simulink model "Bike2DOF"  (R2023a)
settings: Solver=VariableStepAuto  StartTime=0.0  StopTime=10.0  RelTol=1e-3
undefined symbols (not defined in the file): Iz, l_f, l_r, m
settings Model: Creator=Tan_Tram  LastModifiedBy=Tan_Tram

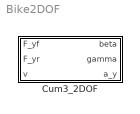
== system Bike2DOF ==
  Cum3_2DOF : Subsystem

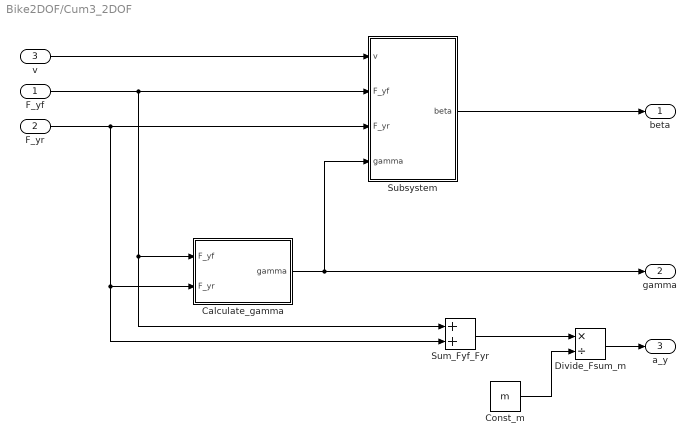
== system Bike2DOF/Cum3_2DOF ==
  F_yf : Inport
  F_yr : Inport  Port=2
  v : Inport  Port=3
  Calculate_gamma : Subsystem
  Const_m : Constant  Value=m
  Divide_Fsum_m : Product  Inputs=*/
  Subsystem : Subsystem
  Sum_Fyf_Fyr : Sum
  beta : Outport
  gamma : Outport  Port=2
  a_y : Outport  Port=3
  wires:
  F_yf/1 -> Subsystem/2(F_yf), Calculate_gamma/1(F_yf), Sum_Fyf_Fyr/1
  F_yr/1 -> Calculate_gamma/2(F_yr), Sum_Fyf_Fyr/2, Subsystem/3(F_yr)
  Const_m/1 -> Divide_Fsum_m/2
  Sum_Fyf_Fyr/1 -> Divide_Fsum_m/1
  Divide_Fsum_m/1 -> a_y/1
  Calculate_gamma/1(gamma) -> Subsystem/4(gamma), gamma/1
  v/1 -> Subsystem/1(v)
  Subsystem/1(beta) -> beta/1

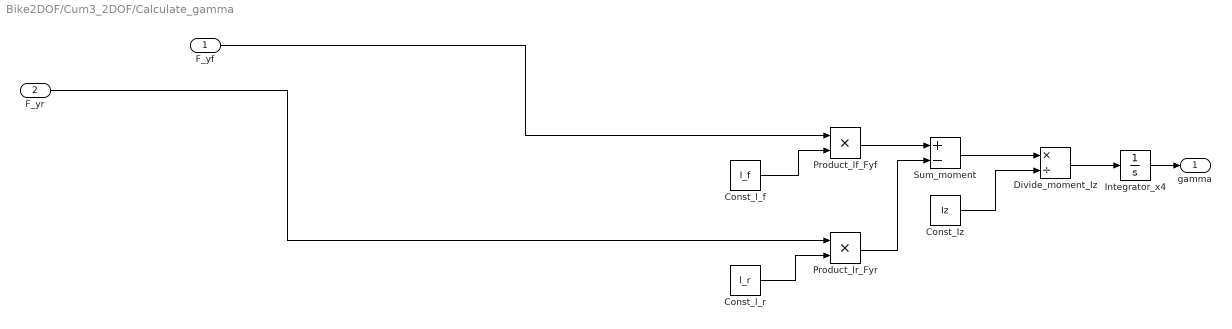
== system Bike2DOF/Cum3_2DOF/Calculate_gamma ==
  F_yf : Inport
  F_yr : Inport  Port=2
  Const_Iz : Constant  Value=Iz
  Const_l_f : Constant  Value=l_f
  Const_l_r : Constant  Value=l_r
  Divide_moment_Iz : Product  Inputs=*/
  Integrator_x4 : Integrator
  Product_lf_Fyf : Product  Inputs=**
  Product_lr_Fyr : Product  Inputs=**
  Sum_moment : Sum  Inputs=+-
  gamma : Outport
  wires:
  Const_l_r/1 -> Product_lr_Fyr/2
  Product_lf_Fyf/1 -> Sum_moment/1
  Divide_moment_Iz/1 -> Integrator_x4/1
  Integrator_x4/1 -> gamma/1
  Const_Iz/1 -> Divide_moment_Iz/2
  Sum_moment/1 -> Divide_moment_Iz/1
  Const_l_f/1 -> Product_lf_Fyf/2
  Product_lr_Fyr/1 -> Sum_moment/2
  F_yf/1 -> Product_lf_Fyf/1
  F_yr/1 -> Product_lr_Fyr/1

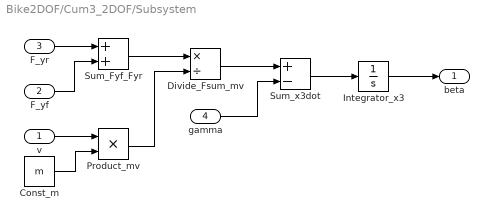
== system Bike2DOF/Cum3_2DOF/Subsystem ==
  v : Inport
  F_yf : Inport  Port=2
  F_yr : Inport  Port=3
  gamma : Inport  Port=4
  Const_m : Constant  Value=m
  Divide_Fsum_mv : Product  Inputs=*/
  Integrator_x3 : Integrator
  Product_mv : Product  Inputs=**
  Sum_Fyf_Fyr : Sum
  Sum_x3dot : Sum  Inputs=+-
  beta : Outport
  wires:
  Product_mv/1 -> Divide_Fsum_mv/2
  Sum_Fyf_Fyr/1 -> Divide_Fsum_mv/1
  F_yf/1 -> Sum_Fyf_Fyr/2
  F_yr/1 -> Sum_Fyf_Fyr/1
  gamma/1 -> Sum_x3dot/2
  Const_m/1 -> Product_mv/2
  v/1 -> Product_mv/1
  Divide_Fsum_mv/1 -> Sum_x3dot/1
  Sum_x3dot/1 -> Integrator_x3/1
  Integrator_x3/1 -> beta/1
